simulink model "Noa_Nofusion"  (R2020b)
settings: Solver=FixedStepDiscrete  StartTime=0.0  StopTime=Inf  FixedStep=0.01  RelTol=1e-3
PostLoadFcn:
  | if any(exist('dsrtsu_mdlpostloadfcn', 'file') ~= 0), dsrtsu_mdlpostloadfcn('Execute', bdroot); end
InitFcn:
  | , if any(exist('rtifpga_mdlclblib', 'file') ~= 0), rtifpga_mdlclblib('Init', bdroot); end,
  | , if any(exist('dsmpb_private', 'file') ~= 0), dsmpb_private('dsmpb_mdlclblib', 'Init', bdroot); end,
undefined symbols (not defined in the file or in its folder): ACC_TimeGap_DecSetSwt, ACC_TimeGap_IncSetSwt, AccelPedalPosn, AccelPedalPosnVldty, AccelPedlPosnDiagc, AccPedalOverride, ACU_ShiftInProgress, ADAS_Posn_CurLane, AESSwtReq, ALC_SwtReq, BrkPedalSts, CC_ACC_CANCEL_OFFSwt, CC_ACC_CRUISE_OFFSwt, CC_ACC_DecSetSpd_SetSwt, CC_ACC_IncSetSpd_ResuSwt, CC_ACCSwtErr, CharSpd_ms, CSA_NODE, CURRENT_GEAR, CurrentGearValid, DiscIntNeverNeededParam, DrvDoorSts, DrvSBR, DrvTrqReqOvld, ECMACCInterface, ECMRespACC, ELKSwtReq, EngLimpHomeSts, EngSpd, EngState, EngState_PHEV, EngTrqMaxActSpd, EngTrqMinAct, EPS_DrvInpTrqVal_HighReslolution, EPS_FailSts, EPS_LKATorqOvrlDlvd, EPS_LKATorqOvrlDlvdVld, EPS_LKATrqOvlDlvdSts, EPS_SteerMod, EPS_TrqSnsrSts, EQ4_APPINFO, EQ4_LA_ELEM, EQ4_LA_HDR, EQ4_LAP_ELEM, EQ4_LAP_HDR, EQ4_LH_ELEM, EQ4_LH_HDR, EQ4_LRE_ELEM, EQ4_LRE_HDR, ESS_PedSwtReq, ESS_VehSwtReq, FFogLmpSts_F_Pbox, FLWheelDriveDirection, FLWheelSpd, FrntWiprSwtSts, FrntWshrSwtSts, FRWheelDriveDirection, FRWheelSpd, HazardLmpSwtSts, HCU_AccelPedalPosn_Diag ... (+151)
libraries: simulink x144, dsmpblib x33, canfdmsglib x10
(part 13 of 20)

== system Noa_Nofusion/Common/Subsystem7/DS/DriverStsConditnJudge/DSMidHi1Hi22NoDistractnJudge ==
  note: %Note
      | In order to cover one case at which distraction is no distraction but drowsns is low/middle/high 1/high2,add this
      | transition from low/middle/high 1/high2 distraction to no distraction.Conditions as follow:
      | DMSSts_ACC is 0x02: Active
      | && HeadDetn is 0x01: Yes
      | && DistrctnLevel_ACC is 0x00: No distraction
      | && DistrctnQlty_ACC≥ 85%
      | && During time is same as time of other to good
  canDMSSts : Inport
  canHeadDetn : Inport  Port=2
  canDistrctnLevel : Inport  Port=3
  canDistrctnQlty : Inport  Port=4
  Compare To Constant : simulink/Logic and Bit Operations/Compare To Constant  relop===  const=2  OutDataTypeStr=boolean
  Compare To Constant1 : simulink/Logic and Bit Operations/Compare To Constant  relop===  const=1  OutDataTypeStr=boolean
  Compare To Constant2 : simulink/Logic and Bit Operations/Compare To Constant  relop===  const=0  OutDataTypeStr=boolean
  Compare To Constant4 : simulink/Logic and Bit Operations/Compare To Constant  relop=>=  const=85  OutDataTypeStr=boolean
  Compare To Constant5 : simulink/Logic and Bit Operations/Compare To Constant  relop=>=  const=0.5  OutDataTypeStr=boolean
  Compare To Constant8 : simulink/Logic and Bit Operations/Compare To Constant  relop=<=  const=100  OutDataTypeStr=boolean
  Data Type Conversion : DataTypeConversion  OutDataTypeStr=single
  Logical Operator : Logic  Inputs=5  AllPortsSameDT=off  OutDataTypeStr=boolean
  counter : DiscreteIntegrator  ExternalReset=either  SampleTime=-1  LimitOutput=on  UpperSaturationLimit=10  LowerSaturationLimit=-10  ICPrevOutput=DiscIntNeverNeededParam  ICPrevScaledInput=DiscIntNeverNeededParam
  DSMidHi1Hi22NoDistractn : Outport
  wires:
  Compare To Constant5/1 -> DSMidHi1Hi22NoDistractn/1
  Compare To Constant8/1 -> Logical Operator/5
  Compare To Constant4/1 -> Logical Operator/4
  Compare To Constant2/1 -> Logical Operator/3
  Compare To Constant/1 -> Logical Operator/1
  Compare To Constant1/1 -> Logical Operator/2
  canDistrctnQlty/1 -> Compare To Constant4/1, Compare To Constant8/1
  counter/1 -> Compare To Constant5/1
  Logical Operator/1 -> Data Type Conversion/1
  canDistrctnLevel/1 -> Compare To Constant2/1
  canHeadDetn/1 -> Compare To Constant1/1
  canDMSSts/1 -> Compare To Constant/1
  Data Type Conversion/1 -> counter/2, counter/1

== system Noa_Nofusion/Common/Subsystem7/DS/DriverStsConditnJudge/DSMidHi1Hi22NoDrowsnsJudge ==
  note: %Note
      | In order to cover one case at which drowsns is no drowsiness but distraction is low/middle/high 1/high2,add this
      | transition from low/middle/high 1/high2 drowsiness to no drowsiness.Conditions as follow:
      | DMSSts_ACC is 0x02: Active
      | && HeadDetn is 0x01: Yes
      | && DrowsnsLevel_ACC is：0x0: No Drowsiness
      | && DrowsnsQlty_ACC≥85%
      | && During time is same as time of other to good
  canDMSSts : Inport
  canHeadDetn : Inport  Port=2
  canDrowsnsLevel : Inport  Port=3
  Compare To Constant : simulink/Logic and Bit Operations/Compare To Constant  relop===  const=2  OutDataTypeStr=boolean
  Compare To Constant1 : simulink/Logic and Bit Operations/Compare To Constant  relop===  const=1  OutDataTypeStr=boolean
  Compare To Constant2 : simulink/Logic and Bit Operations/Compare To Constant  relop===  const=0  OutDataTypeStr=boolean
  Compare To Constant5 : simulink/Logic and Bit Operations/Compare To Constant  relop=>=  const=0.5  OutDataTypeStr=boolean
  Data Type Conversion : DataTypeConversion  OutDataTypeStr=single
  Logical Operator : Logic  Inputs=3  AllPortsSameDT=off  OutDataTypeStr=boolean
  counter : DiscreteIntegrator  ExternalReset=either  SampleTime=-1  LimitOutput=on  UpperSaturationLimit=10  LowerSaturationLimit=-10  ICPrevOutput=DiscIntNeverNeededParam  ICPrevScaledInput=DiscIntNeverNeededParam
  DSMidHi1Hi22NoDrowsns : Outport
  wires:
  canDMSSts/1 -> Compare To Constant/1
  canHeadDetn/1 -> Compare To Constant1/1
  canDrowsnsLevel/1 -> Compare To Constant2/1
  Logical Operator/1 -> Data Type Conversion/1
  counter/1 -> Compare To Constant5/1
  Compare To Constant1/1 -> Logical Operator/2
  Compare To Constant/1 -> Logical Operator/1
  Compare To Constant2/1 -> Logical Operator/3
  Compare To Constant5/1 -> DSMidHi1Hi22NoDrowsns/1
  Data Type Conversion/1 -> counter/2, counter/1

== system Noa_Nofusion/Common/Subsystem7/DS/DriverStsConditnJudge/DSOther2GoodJudge ==
  note: %Note
      | Conditions of distraction state from Unbelievable∥Low∥Middle∥High Level 1∥High Level 2 to Good as follows:
      | DMSSts_ACC is 0x02: Active
      | && HeadDetn is 0x01: Yes
      | && DistrctnLevel_ACC is 0x00: No distraction
      | && DistrctnQlty_ACC≥ 85%
      | && DrowsnsLevel_ACC is：0x0: No Drowsiness
      | && DrowsnsQlty_ACC≥85%
      | && During time≥0.5s
  canDMSSts : Inport
  canHeadDetn : Inport  Port=2
  canDistrctnLevel : Inport  Port=3
  canDistrctnQlty : Inport  Port=4
  canDrowsnsLevel : Inport  Port=5
  Compare To Constant : simulink/Logic and Bit Operations/Compare To Constant  relop===  const=2  OutDataTypeStr=boolean
  Compare To Constant1 : simulink/Logic and Bit Operations/Compare To Constant  relop===  const=1  OutDataTypeStr=boolean
  Compare To Constant2 : simulink/Logic and Bit Operations/Compare To Constant  relop===  const=0  OutDataTypeStr=boolean
  Compare To Constant3 : simulink/Logic and Bit Operations/Compare To Constant  relop=>=  const=85  OutDataTypeStr=boolean
  Compare To Constant4 : simulink/Logic and Bit Operations/Compare To Constant  relop=<=  const=100  OutDataTypeStr=boolean
  Compare To Constant5 : simulink/Logic and Bit Operations/Compare To Constant  relop=>=  const=0.5  OutDataTypeStr=boolean
  Compare To Constant6 : simulink/Logic and Bit Operations/Compare To Constant  relop===  const=0  OutDataTypeStr=boolean
  Data Type Conversion : DataTypeConversion  OutDataTypeStr=single
  Logical Operator : Logic  Inputs=6  AllPortsSameDT=off  OutDataTypeStr=boolean
  counter : DiscreteIntegrator  ExternalReset=either  SampleTime=-1  LimitOutput=on  UpperSaturationLimit=10  LowerSaturationLimit=-10  ICPrevOutput=DiscIntNeverNeededParam  ICPrevScaledInput=DiscIntNeverNeededParam
  DSOther2Good : Outport
  wires:
  canDMSSts/1 -> Compare To Constant/1
  canHeadDetn/1 -> Compare To Constant1/1
  canDistrctnLevel/1 -> Compare To Constant2/1
  canDistrctnQlty/1 -> Compare To Constant4/1, Compare To Constant3/1
  Logical Operator/1 -> Data Type Conversion/1
  counter/1 -> Compare To Constant5/1
  canDrowsnsLevel/1 -> Compare To Constant6/1
  Compare To Constant/1 -> Logical Operator/1
  Compare To Constant1/1 -> Logical Operator/2
  Compare To Constant2/1 -> Logical Operator/3
  Compare To Constant3/1 -> Logical Operator/4
  Compare To Constant4/1 -> Logical Operator/5
  Compare To Constant6/1 -> Logical Operator/6
  Compare To Constant5/1 -> DSOther2Good/1
  Data Type Conversion/1 -> counter/2, counter/1

== system Noa_Nofusion/Common/Subsystem7/DS/DriverStsConditnJudge/DSOther2Hi1DistractnJudge ==
  note: %Note
      | Conditions of distraction state from other state to High 1 as follow:
      | DMSSts_ACC is 0x02: Active
      | && HeadDetn is 0x01: Yes
      | && DistrctnLevel_ACC is 0x03: Hi level distraction
      | && DistrctnQlty_ACC≥ 85%
      | && During time≥2s(adjustable)
  canDMSSts : Inport
  canHeadDetn : Inport  Port=2
  canDistrctnLevel : Inport  Port=3
  canDistrctnQlty : Inport  Port=4
  PtDSOther2Hi1Distractn : Inport  Port=5
  Compare To Constant : simulink/Logic and Bit Operations/Compare To Constant  relop===  const=2  OutDataTypeStr=boolean
  Compare To Constant1 : simulink/Logic and Bit Operations/Compare To Constant  relop===  const=1  OutDataTypeStr=boolean
  Compare To Constant2 : simulink/Logic and Bit Operations/Compare To Constant  relop===  const=3  OutDataTypeStr=boolean
  Compare To Constant4 : simulink/Logic and Bit Operations/Compare To Constant  relop=>=  const=85  OutDataTypeStr=boolean
  Compare To Constant8 : simulink/Logic and Bit Operations/Compare To Constant  relop=<=  const=100  OutDataTypeStr=boolean
  Data Type Conversion : DataTypeConversion  OutDataTypeStr=single
  Logical Operator : Logic  Inputs=5  AllPortsSameDT=off  OutDataTypeStr=boolean
  Relational Operator : RelationalOperator  OutDataTypeStr=boolean  RndMeth=Simplest
  counter : DiscreteIntegrator  ExternalReset=either  SampleTime=-1  LimitOutput=on  UpperSaturationLimit=10  LowerSaturationLimit=-10  ICPrevOutput=DiscIntNeverNeededParam  ICPrevScaledInput=DiscIntNeverNeededParam
  DSOther2Hi1Distractn : Outport
  wires:
  Logical Operator/1 -> Data Type Conversion/1
  canDMSSts/1 -> Compare To Constant/1
  canHeadDetn/1 -> Compare To Constant1/1
  canDistrctnLevel/1 -> Compare To Constant2/1
  canDistrctnQlty/1 -> Compare To Constant8/1, Compare To Constant4/1
  Compare To Constant1/1 -> Logical Operator/2
  Compare To Constant/1 -> Logical Operator/1
  Compare To Constant2/1 -> Logical Operator/3
  Compare To Constant4/1 -> Logical Operator/4
  Compare To Constant8/1 -> Logical Operator/5
  Relational Operator/1 -> DSOther2Hi1Distractn/1
  counter/1 -> Relational Operator/1
  PtDSOther2Hi1Distractn/1 -> Relational Operator/2
  Data Type Conversion/1 -> counter/2, counter/1

== system Noa_Nofusion/Common/Subsystem7/DS/DriverStsConditnJudge/DSOther2Hi1DrowsnsJudge ==
  note: %Note
      | Conditions of drowsns state from other state to High 1 as follow:
      | DMSSts_ACC is 0x02: Active
      | && HeadDetn is 0x01: Yes
      | && DrowsnsLevel_ACC is 0x3: Hi level Drowsiness
      | && DrowsnsQlty_ACC≥85%
      | && During time≥0.5s(adjustable)
  canDMSSts : Inport
  canHeadDetn : Inport  Port=2
  canDrowsnsLevel : Inport  Port=3
  PtDSOther2Hi1Drowsns : Inport  Port=4
  Compare To Constant : simulink/Logic and Bit Operations/Compare To Constant  relop===  const=2  OutDataTypeStr=boolean
  Compare To Constant1 : simulink/Logic and Bit Operations/Compare To Constant  relop===  const=1  OutDataTypeStr=boolean
  Compare To Constant2 : simulink/Logic and Bit Operations/Compare To Constant  relop===  const=3  OutDataTypeStr=boolean
  Data Type Conversion : DataTypeConversion  OutDataTypeStr=single
  Logical Operator : Logic  Inputs=3  AllPortsSameDT=off  OutDataTypeStr=boolean
  Relational Operator : RelationalOperator  OutDataTypeStr=boolean  RndMeth=Simplest
  counter : DiscreteIntegrator  ExternalReset=either  SampleTime=-1  LimitOutput=on  UpperSaturationLimit=10  LowerSaturationLimit=-10  ICPrevOutput=DiscIntNeverNeededParam  ICPrevScaledInput=DiscIntNeverNeededParam
  DSOther2Hi1Drowsns : Outport
  wires:
  counter/1 -> Relational Operator/1
  Relational Operator/1 -> DSOther2Hi1Drowsns/1
  Compare To Constant2/1 -> Logical Operator/3
  Compare To Constant/1 -> Logical Operator/1
  Compare To Constant1/1 -> Logical Operator/2
  canDrowsnsLevel/1 -> Compare To Constant2/1
  canHeadDetn/1 -> Compare To Constant1/1
  canDMSSts/1 -> Compare To Constant/1
  Logical Operator/1 -> Data Type Conversion/1
  PtDSOther2Hi1Drowsns/1 -> Relational Operator/2
  Data Type Conversion/1 -> counter/2, counter/1

== system Noa_Nofusion/Common/Subsystem7/DS/DriverStsConditnJudge/DSOther2Hi2DistractnJudge ==
  note: %Note
      | Conditions of distraction state from other state to High 2 as follow:
      | DMSSts_ACC is 0x02: Active
      | && HeadDetn is 0x01: Yes
      | && DistrctnLevel_ACC is 0x03: Hi level distraction
      | && DistrctnQlty_ACC≥ 85%
      | && During time≥5s(adjustable)
  canDMSSts : Inport
  canHeadDetn : Inport  Port=2
  canDistrctnLevel : Inport  Port=3
  canDistrctnQlty : Inport  Port=4
  PtDSOther2Hi2Distractn : Inport  Port=5
  Compare To Constant : simulink/Logic and Bit Operations/Compare To Constant  relop===  const=2  OutDataTypeStr=boolean
  Compare To Constant1 : simulink/Logic and Bit Operations/Compare To Constant  relop===  const=1  OutDataTypeStr=boolean
  Compare To Constant2 : simulink/Logic and Bit Operations/Compare To Constant  relop===  const=3  OutDataTypeStr=boolean
  Compare To Constant4 : simulink/Logic and Bit Operations/Compare To Constant  relop=>=  const=85  OutDataTypeStr=boolean
  Compare To Constant8 : simulink/Logic and Bit Operations/Compare To Constant  relop=<=  const=100  OutDataTypeStr=boolean
  Data Type Conversion : DataTypeConversion  OutDataTypeStr=single
  Logical Operator : Logic  Inputs=5  AllPortsSameDT=off  OutDataTypeStr=boolean
  Relational Operator : RelationalOperator  OutDataTypeStr=boolean  RndMeth=Simplest
  counter : DiscreteIntegrator  ExternalReset=either  SampleTime=-1  LimitOutput=on  UpperSaturationLimit=10  LowerSaturationLimit=-10  ICPrevOutput=DiscIntNeverNeededParam  ICPrevScaledInput=DiscIntNeverNeededParam
  DSOther2Hi2Distractn : Outport
  wires:
  counter/1 -> Relational Operator/1
  Relational Operator/1 -> DSOther2Hi2Distractn/1
  Compare To Constant8/1 -> Logical Operator/5
  Compare To Constant4/1 -> Logical Operator/4
  Compare To Constant2/1 -> Logical Operator/3
  Compare To Constant/1 -> Logical Operator/1
  Compare To Constant1/1 -> Logical Operator/2
  canDistrctnQlty/1 -> Compare To Constant4/1, Compare To Constant8/1
  canDistrctnLevel/1 -> Compare To Constant2/1
  canHeadDetn/1 -> Compare To Constant1/1
  canDMSSts/1 -> Compare To Constant/1
  Logical Operator/1 -> Data Type Conversion/1
  PtDSOther2Hi2Distractn/1 -> Relational Operator/2
  Data Type Conversion/1 -> counter/2, counter/1

== system Noa_Nofusion/Common/Subsystem7/DS/DriverStsConditnJudge/DSOther2Hi2DrowsnsJudge ==
  note: %Note
      | Conditions of drowsns state from other state to High2 as follow:
      | DMSSts_ACC is 0x02: Active
      | && HeadDetn is 0x01: Yes
      | && DrowsnsLevel_ACC is 0x3: Hi level Drowsiness
      | && DrowsnsQlty_ACC≥85%
      | && During time≥3s(adjustable)
  canDMSSts : Inport
  canHeadDetn : Inport  Port=2
  canDrowsnsLevel : Inport  Port=3
  PtDSOther2Hi2Drowsns : Inport  Port=4
  Compare To Constant : simulink/Logic and Bit Operations/Compare To Constant  relop===  const=2  OutDataTypeStr=boolean
  Compare To Constant1 : simulink/Logic and Bit Operations/Compare To Constant  relop===  const=1  OutDataTypeStr=boolean
  Compare To Constant2 : simulink/Logic and Bit Operations/Compare To Constant  relop===  const=3  OutDataTypeStr=boolean
  Data Type Conversion : DataTypeConversion  OutDataTypeStr=single
  Logical Operator : Logic  Inputs=3  AllPortsSameDT=off  OutDataTypeStr=boolean
  Relational Operator : RelationalOperator  OutDataTypeStr=boolean  RndMeth=Simplest
  counter : DiscreteIntegrator  ExternalReset=either  SampleTime=-1  LimitOutput=on  UpperSaturationLimit=10  LowerSaturationLimit=-10  ICPrevOutput=DiscIntNeverNeededParam  ICPrevScaledInput=DiscIntNeverNeededParam
  DSOther2Hi2Drowsns : Outport
  wires:
  Logical Operator/1 -> Data Type Conversion/1
  canDMSSts/1 -> Compare To Constant/1
  canHeadDetn/1 -> Compare To Constant1/1
  canDrowsnsLevel/1 -> Compare To Constant2/1
  Relational Operator/1 -> DSOther2Hi2Drowsns/1
  Compare To Constant1/1 -> Logical Operator/2
  Compare To Constant/1 -> Logical Operator/1
  Compare To Constant2/1 -> Logical Operator/3
  counter/1 -> Relational Operator/1
  PtDSOther2Hi2Drowsns/1 -> Relational Operator/2
  Data Type Conversion/1 -> counter/2, counter/1

== system Noa_Nofusion/Common/Subsystem7/DS/DriverStsConditnJudge/DSOther2UnbelivJudge ==
  note: %Note
      | Conditions of distraction and drowsns state from other to unbelievable as follow:
      | (DMSSts_ACC is no 0x02: Active&& during time ≥3cycles)
      | ∥ (HeadDetn is 0x00: No&&during time≥3s)
      | ∥(DistrctnLevel_ACC is 0x7: Invalid &&during time≥3s)
      | ∥(DrowsnsLevel_ACC is 0x7: Invalid &&during time≥3s)
      | ∥{DistrctnQlty_ACC is 0x7F:Invalid data &&during time≥3s}
      | ∥{DrowsnsQlty_ACC is 0x7F:Invalid data &&during time≥3s}
  canDMSSts : Inport
  canHeadDetn : Inport  Port=2
  canDistrctnLevel : Inport  Port=3
  canDistrctnQlty : Inport  Port=4
  canDrowsnsLevel : Inport  Port=5
  Compare To Constant : simulink/Logic and Bit Operations/Compare To Constant  relop=~=  const=2  OutDataTypeStr=boolean
  Compare To Constant1 : simulink/Logic and Bit Operations/Compare To Constant  relop===  const=0  OutDataTypeStr=boolean
  Compare To Constant{4,9..11} (4 alike) : simulink/Logic and Bit Operations/Compare To Constant  relop=>=  const=3  OutDataTypeStr=boolean
  Compare To Constant2 : simulink/Logic and Bit Operations/Compare To Constant  relop===  const=7  OutDataTypeStr=boolean
  Compare To Constant3 : simulink/Logic and Bit Operations/Compare To Constant  relop===  const=127  OutDataTypeStr=boolean
  Compare To Constant6 : simulink/Logic and Bit Operations/Compare To Constant  relop===  const=7  OutDataTypeStr=boolean
  Data Type Conversion{,1..4} (5 alike) : DataTypeConversion  OutDataTypeStr=single
  Logical Operator : Logic  Operator=OR  Inputs=5  AllPortsSameDT=off  OutDataTypeStr=boolean
  counter{,1..4} (5 alike) : DiscreteIntegrator  ExternalReset=either  SampleTime=-1  LimitOutput=on  UpperSaturationLimit=10  LowerSaturationLimit=-10  ICPrevOutput=DiscIntNeverNeededParam  ICPrevScaledInput=DiscIntNeverNeededParam
  tCycle3plus : simulink/Logic and Bit Operations/Compare To Constant  relop=>=  const=0.06  OutDataTypeStr=boolean
  DSOther2Unbeliv : Outport
  wires:
  Logical Operator/1 -> DSOther2Unbeliv/1
  canDrowsnsLevel/1 -> Compare To Constant6/1
  canDistrctnQlty/1 -> Compare To Constant3/1
  canDistrctnLevel/1 -> Compare To Constant2/1
  canHeadDetn/1 -> Compare To Constant1/1
  canDMSSts/1 -> Compare To Constant/1
  Compare To Constant1/1 -> Data Type Conversion1/1
  Compare To Constant2/1 -> Data Type Conversion2/1
  Compare To Constant6/1 -> Data Type Conversion3/1
  Compare To Constant3/1 -> Data Type Conversion4/1
  Compare To Constant10/1 -> Logical Operator/3
  Compare To Constant11/1 -> Logical Operator/4
  Compare To Constant9/1 -> Logical Operator/2
  Compare To Constant4/1 -> Logical Operator/5
  tCycle3plus/1 -> Logical Operator/1
  Compare To Constant/1 -> Data Type Conversion/1
  counter/1 -> tCycle3plus/1
  counter1/1 -> Compare To Constant9/1
  counter2/1 -> Compare To Constant10/1
  counter3/1 -> Compare To Constant11/1
  counter4/1 -> Compare To Constant4/1
  Data Type Conversion/1 -> counter/2, counter/1
  Data Type Conversion1/1 -> counter1/2, counter1/1
  Data Type Conversion2/1 -> counter2/2, counter2/1
  Data Type Conversion3/1 -> counter3/2, counter3/1
  Data Type Conversion4/1 -> counter4/2, counter4/1

== system Noa_Nofusion/Common/Subsystem7/DS/DriverStsConditnJudge/DSUnbeliv2DDAJudge ==
  note: %Note
      | Following condition aims to prevent transition between DDA and Unbelievable constantly
      | DMSSts_ACC is 0x02: Active&&
      | HeadDetn is 0x01: Yes &&
      | DistrctnLevel_ACC is no 0x7: Invalid&&
      | DrowsnsLevel_ACC is no 0x7: Invalid&&
      | DistrctnQlty_ACC is no 0x7F:Invalid&&
      | DrowsnsQlty_ACC is no 0x7F:Invalid
  canDMSSts : Inport
  canHeadDetn : Inport  Port=2
  canDistrctnLevel : Inport  Port=3
  canDistrctnQlty : Inport  Port=4
  canDrowsnsLevel : Inport  Port=5
  Compare To Constant : simulink/Logic and Bit Operations/Compare To Constant  relop===  const=2  OutDataTypeStr=boolean
  Compare To Constant1 : simulink/Logic and Bit Operations/Compare To Constant  relop===  const=1  OutDataTypeStr=boolean
  Compare To Constant2 : simulink/Logic and Bit Operations/Compare To Constant  relop=~=  const=7  OutDataTypeStr=boolean
  Compare To Constant3 : simulink/Logic and Bit Operations/Compare To Constant  relop=~=  const=127  OutDataTypeStr=boolean
  Compare To Constant6 : simulink/Logic and Bit Operations/Compare To Constant  relop=~=  const=7  OutDataTypeStr=boolean
  Logical Operator : Logic  Inputs=5  AllPortsSameDT=off  OutDataTypeStr=boolean
  DSUnbeliv2DDAEnable : Outport
  wires:
  canDMSSts/1 -> Compare To Constant/1
  canHeadDetn/1 -> Compare To Constant1/1
  canDistrctnLevel/1 -> Compare To Constant2/1
  canDistrctnQlty/1 -> Compare To Constant3/1
  canDrowsnsLevel/1 -> Compare To Constant6/1
  Logical Operator/1 -> DSUnbeliv2DDAEnable/1
  Compare To Constant/1 -> Logical Operator/1
  Compare To Constant1/1 -> Logical Operator/2
  Compare To Constant2/1 -> Logical Operator/3
  Compare To Constant6/1 -> Logical Operator/4
  Compare To Constant3/1 -> Logical Operator/5

== system Noa_Nofusion/TOS/Subsystem2/ACCOSM/HWA_Task100ms1/OTL1 ==
  vRef : Inport
  tCycle : Inport  Port=2
  tSameHandle : Inport  Port=3
  CutIn : Inport  Port=4
  P0Dx : Inport  Port=5
  P0Dy : Inport  Port=6
  EgoDDeltaX : Inport  Port=7
  EgoDDeltaY : Inport  Port=8
  EgoCosOfPsi : Inport  Port=9
  EgoSinOfPsi : Inport  Port=10
  TarLineValid : Inport  Port=11
  TarLineA2 : Inport  Port=12
  TarLineA1 : Inport  Port=13
  TarLineA0 : Inport  Port=14
  Abs : Abs
  CutIn1 : InportShadow  Port=4
  Logical Operator : Logic  AllPortsSameDT=off  OutDataTypeStr=boolean
  Logical Operator1 : Logic  AllPortsSameDT=off  OutDataTypeStr=boolean
  MATLAB Function : MATLAB Function  TreatAsAtomicUnit=on
  Memory31 : Memory  InitialCondition=zeros(24,1)  InheritSampleTime=on
  Memory32 : Memory  InitialCondition=zeros(24,1)  InheritSampleTime=on
  Memory33 : Memory  InitialCondition=uint8(0)  InheritSampleTime=on
  P0TrajHistCalc01 : MATLAB Function  TreatAsAtomicUnit=on
  P0TrajHistCalc1 : MATLAB Function  TreatAsAtomicUnit=on
  Terminator : Terminator
  Terminator1 : Terminator
  Terminator2 : Terminator
  Unit Delay : UnitDelay  SampleTime=-1  HasFrameUpgradeWarning=on
  tSameHandle1 : InportShadow  Port=3
  LineValid : Outport
  a : Outport  Port=2
  b : Outport  Port=3
  c : Outport  Port=4
  d : Outport  Port=5
  dxMin : Outport  Port=6
  dxMax : Outport  Port=7
  wires:
  vRef/1 -> P0TrajHistCalc01/1(vRef)
  CutIn/1 -> P0TrajHistCalc01/4(CutIn)
  P0TrajHistCalc1/8(d) -> d/1
  P0TrajHistCalc1/10(dxMax) -> dxMax/1
  P0TrajHistCalc1/9(dxMin) -> dxMin/1
  P0TrajHistCalc1/7(c) -> c/1
  P0TrajHistCalc1/6(b) -> b/1
  P0TrajHistCalc1/5(a) -> a/1
  P0TrajHistCalc1/4(LineValid) -> Logical Operator/2
  P0TrajHistCalc1/3(P0TrajHistDyv) -> Terminator2/1
  P0TrajHistCalc1/2(P0TrajHistDxv) -> Terminator1/1
  P0TrajHistCalc1/1(P0TrajHistNum) -> Terminator/1
  P0Dy/1 -> P0TrajHistCalc01/6(P0Dy)
  P0Dx/1 -> P0TrajHistCalc01/5(P0Dx)
  tSameHandle/1 -> P0TrajHistCalc01/3(tSameHandle)
  EgoCosOfPsi/1 -> P0TrajHistCalc01/9(EgoCosOfPsi)
  tCycle/1 -> P0TrajHistCalc01/2(tCycle)
  Memory31/1 -> P0TrajHistCalc01/17(P0TrajHistDyvK1)
  EgoDDeltaY/1 -> P0TrajHistCalc01/8(EgoDDeltaY)
  P0TrajHistCalc01/3(P0TrajHistDxv) -> P0TrajHistCalc1/2(P0TrajHistDxv1), Memory32/1
  Memory32/1 -> P0TrajHistCalc01/16(P0TrajHistDxvK1)
  P0TrajHistCalc01/2(P0TrajHistNum) -> P0TrajHistCalc1/1(P0TrajHistNum1), Memory33/1
  EgoSinOfPsi/1 -> P0TrajHistCalc01/10(EgoSinOfPsi)
  Memory33/1 -> P0TrajHistCalc01/15(P0TrajHistNumK1)
  P0TrajHistCalc01/4(P0TrajHistDyv) -> P0TrajHistCalc1/3(P0TrajHistDyv1), Memory31/1
  EgoDDeltaX/1 -> P0TrajHistCalc01/7(EgoDDeltaX)
  TarLineValid/1 -> P0TrajHistCalc01/11(TarLineValid)
  TarLineA2/1 -> P0TrajHistCalc01/12(TarLineA2)
  TarLineA1/1 -> P0TrajHistCalc01/13(TarLineA1)
  TarLineA0/1 -> P0TrajHistCalc01/14(TarLineA0)
  tSameHandle1/1 -> MATLAB Function/1(t)
  CutIn1/1 -> Logical Operator1/1
  MATLAB Function/1(Valid) -> Logical Operator/1, Unit Delay/1
  Unit Delay/1 -> MATLAB Function/3(ValidK1)
  Logical Operator/1 -> LineValid/1
  P0TrajHistCalc01/1(P0Dyc) -> Abs/1
  Abs/1 -> Logical Operator1/2
  Logical Operator1/1 -> MATLAB Function/2(CutIn_b)

== system Noa_Nofusion/TOS/Subsystem2/ACCOSM/HWA_Task100ms1/Trajectory ==
  Kap : Inport
  VxvRef : Inport  Port=2
  AlpSideSlipAngle : Inport  Port=3
  ObjValid : Inport  Port=4
  ObjDx : Inport  Port=5
  ObjDy : Inport  Port=6
  ObjClass : Inport  Port=7
  ObjCntAlive : Inport  Port=8
  Terminator{1,3..10} (9 alike) : Terminator
  Trajectory : Subsystem  mask{ObjNum=15, TrajNum=10, BufNum=24}
      mask prompts: ObjNum "ObjectNumber"; TrajNum "TrajectoryNumber"; BufNum "BufferNumber"
  Out8 : Outport
  Out9 : Outport  Port=2
  Out10 : Outport  Port=3
  Out11 : Outport  Port=4
  Out12 : Outport  Port=5
  Out13 : Outport  Port=6
  EgoMove : Outport  Port=7
  wires:
  Trajectory/16(EgoMove) -> EgoMove/1
  Trajectory/11(TrajHistBufferBValid) -> Out11/1
  Trajectory/12(TrajHistBufferDxv) -> Out12/1
  Trajectory/13(TrajHistBufferDyv) -> Out13/1
  ObjValid/1 -> Trajectory/4(ObjValid)
  ObjDx/1 -> Trajectory/5(ObjectDx)
  ObjDy/1 -> Trajectory/6(ObjectDy)
  ObjClass/1 -> Trajectory/7(ObjectClass)
  ObjCntAlive/1 -> Trajectory/8(ObjectCntAlive)
  Kap/1 -> Trajectory/1(KapTraj)
  Trajectory/8(TrajHistBufferBTrajEnd) -> Out8/1
  Trajectory/2(EgoTrajHistDxv) -> Terminator4/1
  Trajectory/5(ObjPrio) -> Terminator8/1
  Trajectory/1(EgoTrajHistCurrentIndex) -> Terminator3/1
  AlpSideSlipAngle/1 -> Trajectory/3(AlpSideSlipAngle)
  Trajectory/7(TrajUsed) -> Terminator9/1
  Trajectory/10(TrajCurrentIndex) -> Out10/1
  Trajectory/6(ObjMatrix) -> Terminator10/1
  Trajectory/4(EgoTrajHistTTimeStamp) -> Terminator7/1
  VxvRef/1 -> Trajectory/2(VxvRef)
  Trajectory/3(EgoTrajHistDyv) -> Terminator5/1
  Trajectory/9(ObjTrajNumber) -> Out9/1
  Trajectory/14(TrajHistBufferTTimeStamp) -> Terminator6/1
  Trajectory/15(TrajHistBufferClass) -> Terminator1/1

== system Noa_Nofusion/TOS/Subsystem2/ACCOSM/HWA_Task100ms1/VxVy ==
  VxvRef : Inport
  Kap : Inport  Port=2
  VxG : Inport  Port=3
  VyG : Inport  Port=4
  Constant2 : Constant  Value=P_Global_EQ2RearAxisX_m  OutDataTypeStr=single
  Constant4 : Constant  Value=SideSlipAnglefactor  OutDataTypeStr=single
  Divide11 : Product
  Divide3 : Product  Inputs=3
  Divide4 : Product
  Divide5 : Product
  Gain10 : Gain  Gain=-1
  Gain9 : Gain  Gain=-1
  Sum1 : Sum  Inputs=+-
  Sum10 : Sum  Inputs=+-|
  Sum11 : Sum  Inputs=|-+
  Trigonometric Function : Trigonometry  Operator=atan  OutputSignalType=real
  Trigonometric Function1 : Trigonometry  Operator=cos
  Trigonometric Function2 : Trigonometry
  Vx : Outport
  Vy : Outport  Port=2
  wires:
  VxvRef/1 -> Divide3/2, Divide11/1, Divide5/1, Divide3/3
  Constant4/1 -> Divide3/1
  Trigonometric Function/1 -> Gain9/1
  Divide11/1 -> Sum11/1
  Constant2/1 -> Sum1/1
  Trigonometric Function1/1 -> Divide5/2
  Divide4/1 -> Trigonometric Function/1
  Divide5/1 -> Sum10/2
  Gain10/1 -> Trigonometric Function1/1, Trigonometric Function2/1
  Divide3/1 -> Sum1/2
  [IFVMoveAngle] -> Gain10/1
  Trigonometric Function2/1 -> Divide11/2
  Sum1/1 -> Divide4/1
  Gain9/1 -> [IFVMoveAngle]
  VxG/1 -> Sum10/1
  Sum11/1 -> Vy/1  "Vy"
  Sum10/1 -> Vx/1  "Vx"
  VyG/1 -> Sum11/2
  Kap/1 -> Divide4/2

== system Noa_Nofusion/TOS/Subsystem2/ACCOSM/ObjMatrixTransit/Subsystem ==
  Count : Inport
  <EQ4_OBJ_ELEM> : Inport  Port=2
  Bus Creator : BusCreator  Inputs=12
  Bus Selector : BusSelector  OutputSignals=id,BrakeLight,classification,LatDis,AbsLatVel,AbsLongAcc,LongDis,AbsLongVel,width,Age,motionSts
  For Each Subsystem : Subsystem  TreatAsAtomicUnit=on
  For Iterator Subsystem : Subsystem  Commented=on  TreatAsAtomicUnit=on
  MATLAB Function1 : MATLAB Function  TreatAsAtomicUnit=on
  Obj : Stateflow chart  Commented=on  TreatAsAtomicUnit=on
  Terminator : Terminator
  Terminator1 : Terminator
  Unit Delay1 : UnitDelay  SampleTime=-1  HasFrameUpgradeWarning=on
  ObjID : Outport
  ObjValid : Outport  Port=2
  ObjBrakeLightIndic : Outport  Port=3
  ObjClassification : Outport  Port=4
  ObjLatPos : Outport  Port=5
  ObjLatVel : Outport  Port=6
  ObjLongAccel : Outport  Port=7
  ObjLongVel : Outport  Port=8
  ObjWidth : Outport  Port=9
  ObjCnt : Outport  Port=10
  ObjMoveSts : Outport  Port=11
  ObjLongPos : Outport  Port=12
  P : Outport  Port=13
  ObjClass : Outport  Port=14
  wires:
  For Each Subsystem/6(LatDis) -> Bus Creator/6  "LatDis"
  Bus Creator/1 -> Bus Selector/1
  MATLAB Function1/14(ObjID) -> ObjID/1, Unit Delay1/1  "ObjBrakeLightIndic"
  For Each Subsystem/10(BrakeLight) -> Bus Creator/10  "BrakeLight"
  MATLAB Function1/6(ObjLatPos) -> ObjLatPos/1
  For Each Subsystem/7(AbsLongAcc) -> Bus Creator/7  "AbsLongAcc"
  For Each Subsystem/12(motionSts) -> Bus Creator/12  "motionSts"
  MATLAB Function1/5(ObjClassification) -> ObjClassification/1
  MATLAB Function1/8(ObjLongAccel) -> ObjLongAccel/1
  For Each Subsystem/14(motionOrientation) -> Terminator1/1
  Count/1 -> MATLAB Function1/1(Count)
  For Each Subsystem/8(AbsLongVel) -> Bus Creator/8  "AbsLongVel"
  For Each Subsystem/4(width) -> Bus Creator/4  "width"
  For Each Subsystem/13(motionCategory) -> Terminator/1
  For Each Subsystem/9(AbsLatVel) -> Bus Creator/9  "AbsLatVel"
  For Each Subsystem/5(LongDis) -> Bus Creator/5  "LongDis"
  Bus Selector/10 -> MATLAB Function1/11(Age)  "<Age>"
  For Each Subsystem/3(classification) -> Bus Creator/3  "classification"
  Bus Selector/8 -> MATLAB Function1/9(LongVel)  "<AbsLongVel>"
  Bus Selector/3 -> MATLAB Function1/4(Class)  "<classification>"
  For Each Subsystem/1(id) -> Bus Creator/1  "id"
  For Each Subsystem/11(Age) -> Bus Creator/11  "Age"
  For Each Subsystem/2(confidence) -> Bus Creator/2  "confidence"
  Bus Selector/7 -> MATLAB Function1/8(LongDis)  "<LongDis>"
  Bus Selector/9 -> MATLAB Function1/10(Width)  "<width>"
  Bus Selector/5 -> MATLAB Function1/6(LatVel)  "<AbsLatVel>"
  Bus Selector/6 -> MATLAB Function1/7(LongAccel)  "<AbsLongAcc>"
  Bus Selector/4 -> MATLAB Function1/5(LatDis)  "<LatDis>"
  MATLAB Function1/12(ObjMoveSts) -> ObjMoveSts/1
  Bus Selector/11 -> MATLAB Function1/12(MotionSts)  "<motionSts>"
  MATLAB Function1/13(ObjLongPos) -> ObjLongPos/1
  MATLAB Function1/1(P) -> P/1
  Bus Selector/2 -> MATLAB Function1/3(BrakeLight_b)  "<BrakeLight>"
  Bus Selector/1 -> MATLAB Function1/2(ID)  "<id>"
  Unit Delay1/1 -> MATLAB Function1/13(ObjIDK1)
  <EQ4_OBJ_ELEM>/1 -> For Each Subsystem/1(<EQ4_OBJ_ELEM>)
  MATLAB Function1/2(ObjValid) -> ObjValid/1
  MATLAB Function1/7(ObjLatVel) -> ObjLatVel/1
  MATLAB Function1/3(ObjBrakeLightIndic) -> ObjBrakeLightIndic/1
  MATLAB Function1/9(ObjLongVel) -> ObjLongVel/1
  MATLAB Function1/10(ObjWidth) -> ObjWidth/1
  MATLAB Function1/11(ObjCnt) -> ObjCnt/1
  MATLAB Function1/4(ObjClass) -> ObjClass/1

== system Noa_Nofusion/TOS/Subsystem2/DOP/HWA_Task100ms1/OTL1 ==
  vRef : Inport
  tCycle : Inport  Port=2
  tSameHandle : Inport  Port=3
  CutIn : Inport  Port=4
  P0Dx : Inport  Port=5
  P0Dy : Inport  Port=6
  EgoDDeltaX : Inport  Port=7
  EgoDDeltaY : Inport  Port=8
  EgoCosOfPsi : Inport  Port=9
  EgoSinOfPsi : Inport  Port=10
  TarLineValid : Inport  Port=11
  TarLineA2 : Inport  Port=12
  TarLineA1 : Inport  Port=13
  TarLineA0 : Inport  Port=14
  Memory31 : Memory  InitialCondition=zeros(24,1)  InheritSampleTime=on
  Memory32 : Memory  InitialCondition=zeros(24,1)  InheritSampleTime=on
  Memory33 : Memory  InitialCondition=uint8(0)  InheritSampleTime=on
  P0TrajHistCalc01 : MATLAB Function  TreatAsAtomicUnit=on
  P0TrajHistCalc1 : MATLAB Function  TreatAsAtomicUnit=on
  Terminator{,1..3} (4 alike) : Terminator
  LineValid : Outport
  a : Outport  Port=2
  b : Outport  Port=3
  c : Outport  Port=4
  d : Outport  Port=5
  dxMin : Outport  Port=6
  dxMax : Outport  Port=7
  wires:
  P0TrajHistCalc01/1(P0Dyc) -> Terminator3/1
  P0TrajHistCalc1/4(LineValid) -> LineValid/1
  TarLineA0/1 -> P0TrajHistCalc01/14(TarLineA0)
  TarLineA1/1 -> P0TrajHistCalc01/13(TarLineA1)
  TarLineA2/1 -> P0TrajHistCalc01/12(TarLineA2)
  TarLineValid/1 -> P0TrajHistCalc01/11(TarLineValid)
  EgoDDeltaX/1 -> P0TrajHistCalc01/7(EgoDDeltaX)
  P0TrajHistCalc01/4(P0TrajHistDyv) -> Memory31/1, P0TrajHistCalc1/3(P0TrajHistDyv1)
  Memory33/1 -> P0TrajHistCalc01/15(P0TrajHistNumK1)
  EgoSinOfPsi/1 -> P0TrajHistCalc01/10(EgoSinOfPsi)
  P0TrajHistCalc01/2(P0TrajHistNum) -> Memory33/1, P0TrajHistCalc1/1(P0TrajHistNum1)
  Memory32/1 -> P0TrajHistCalc01/16(P0TrajHistDxvK1)
  P0TrajHistCalc01/3(P0TrajHistDxv) -> Memory32/1, P0TrajHistCalc1/2(P0TrajHistDxv1)
  EgoDDeltaY/1 -> P0TrajHistCalc01/8(EgoDDeltaY)
  Memory31/1 -> P0TrajHistCalc01/17(P0TrajHistDyvK1)
  tCycle/1 -> P0TrajHistCalc01/2(tCycle)
  EgoCosOfPsi/1 -> P0TrajHistCalc01/9(EgoCosOfPsi)
  tSameHandle/1 -> P0TrajHistCalc01/3(tSameHandle)
  P0Dx/1 -> P0TrajHistCalc01/5(P0Dx)
  P0Dy/1 -> P0TrajHistCalc01/6(P0Dy)
  P0TrajHistCalc1/1(P0TrajHistNum) -> Terminator/1
  P0TrajHistCalc1/2(P0TrajHistDxv) -> Terminator1/1
  P0TrajHistCalc1/3(P0TrajHistDyv) -> Terminator2/1
  P0TrajHistCalc1/5(a) -> a/1
  P0TrajHistCalc1/6(b) -> b/1
  P0TrajHistCalc1/7(c) -> c/1
  P0TrajHistCalc1/9(dxMin) -> dxMin/1
  P0TrajHistCalc1/10(dxMax) -> dxMax/1
  P0TrajHistCalc1/8(d) -> d/1
  CutIn/1 -> P0TrajHistCalc01/4(CutIn)
  vRef/1 -> P0TrajHistCalc01/1(vRef)

== system Noa_Nofusion/TOS/Subsystem2/DOP/HWA_Task100ms1/Trajectory ==
  Kap : Inport
  VxvRef : Inport  Port=2
  AlpSideSlipAngle : Inport  Port=3
  ObjValid : Inport  Port=4
  ObjDx : Inport  Port=5
  ObjDy : Inport  Port=6
  ObjClass : Inport  Port=7
  ObjCntAlive : Inport  Port=8
  Terminator{1,3..10} (9 alike) : Terminator
  Trajectory : Subsystem  mask{ObjNum=15, TrajNum=10, BufNum=24}
      mask prompts: ObjNum "ObjectNumber"; TrajNum "TrajectoryNumber"; BufNum "BufferNumber"
  Out8 : Outport
  Out9 : Outport  Port=2
  Out10 : Outport  Port=3
  Out11 : Outport  Port=4
  Out12 : Outport  Port=5
  Out13 : Outport  Port=6
  EgoMove : Outport  Port=7
  wires:
  Trajectory/15(TrajHistBufferClass) -> Terminator1/1
  Trajectory/14(TrajHistBufferTTimeStamp) -> Terminator6/1
  Trajectory/9(ObjTrajNumber) -> Out9/1
  Trajectory/3(EgoTrajHistDyv) -> Terminator5/1
  VxvRef/1 -> Trajectory/2(VxvRef)
  Trajectory/4(EgoTrajHistTTimeStamp) -> Terminator7/1
  Trajectory/6(ObjMatrix) -> Terminator10/1
  Trajectory/10(TrajCurrentIndex) -> Out10/1
  Trajectory/7(TrajUsed) -> Terminator9/1
  AlpSideSlipAngle/1 -> Trajectory/3(AlpSideSlipAngle)
  Trajectory/1(EgoTrajHistCurrentIndex) -> Terminator3/1
  Trajectory/5(ObjPrio) -> Terminator8/1
  Trajectory/2(EgoTrajHistDxv) -> Terminator4/1
  Trajectory/8(TrajHistBufferBTrajEnd) -> Out8/1
  Kap/1 -> Trajectory/1(KapTraj)
  ObjCntAlive/1 -> Trajectory/8(ObjectCntAlive)
  ObjClass/1 -> Trajectory/7(ObjectClass)
  ObjDy/1 -> Trajectory/6(ObjectDy)
  ObjDx/1 -> Trajectory/5(ObjectDx)
  ObjValid/1 -> Trajectory/4(ObjValid)
  Trajectory/13(TrajHistBufferDyv) -> Out13/1
  Trajectory/12(TrajHistBufferDxv) -> Out12/1
  Trajectory/11(TrajHistBufferBValid) -> Out11/1
  Trajectory/16(EgoMove) -> EgoMove/1

== system Noa_Nofusion/TOS/Subsystem2/DOP/HWA_Task100ms1/VxVy ==
  VxvRef : Inport
  Kap : Inport  Port=2
  VxG : Inport  Port=3
  VyG : Inport  Port=4
  Constant2 : Constant  Value=P_Global_EQ2RearAxisX_m  OutDataTypeStr=single
  Constant4 : Constant  Value=SideSlipAnglefactor  OutDataTypeStr=single
  Divide11 : Product
  Divide3 : Product  Inputs=3
  Divide4 : Product
  Divide5 : Product
  Gain10 : Gain  Gain=-1
  Gain9 : Gain  Gain=-1
  Sum1 : Sum  Inputs=+-
  Sum10 : Sum  Inputs=+-|
  Sum11 : Sum  Inputs=|-+
  Trigonometric Function : Trigonometry  Operator=atan  OutputSignalType=real
  Trigonometric Function1 : Trigonometry  Operator=cos
  Trigonometric Function2 : Trigonometry
  Vx : Outport
  Vy : Outport  Port=2
  wires:
  Kap/1 -> Divide4/2
  VyG/1 -> Sum11/2
  Sum10/1 -> Vx/1  "Vx"
  Sum11/1 -> Vy/1  "Vy"
  VxG/1 -> Sum10/1
  Gain9/1 -> [IFVMoveAngle]
  Sum1/1 -> Divide4/1
  Trigonometric Function2/1 -> Divide11/2
  [IFVMoveAngle] -> Gain10/1
  Divide3/1 -> Sum1/2
  Gain10/1 -> Trigonometric Function2/1, Trigonometric Function1/1
  Divide5/1 -> Sum10/2
  Divide4/1 -> Trigonometric Function/1
  Trigonometric Function1/1 -> Divide5/2
  Constant2/1 -> Sum1/1
  Divide11/1 -> Sum11/1
  Trigonometric Function/1 -> Gain9/1
  Constant4/1 -> Divide3/1
  VxvRef/1 -> Divide3/3, Divide5/1, Divide11/1, Divide3/2

== system Noa_Nofusion/TOS/Subsystem2/ObjMatrixTransit/Subsystem/For Each Subsystem ==
  <EQ4_OBJ_ELEM> : Inport  Partition=on  PartitionDimension=1  PartitionWidth=1  PartitionOffset=0
  Bus Selector : BusSelector  OutputSignals=OBJ_ID,OBJ_Existence_Probability,OBJ_Object_Class,OBJ_Width,OBJ_Long_Distance,OBJ_Lat_Distance,OBJ_Abs_Long_Acc,OBJ_Abs_Long_Velocity,OBJ_Abs_Lat_Velocity,OBJ_Brake_Light,OBJ_Object_Age,OBJ_Motion_Status,OBJ_Motion_Category,OBJ_Motion_Orientation
  For Each : ForEach  DisableCoverage=on
  id : Outport  ConcatenationDimension=1
  confidence : Outport  Port=2  ConcatenationDimension=1
  classification : Outport  Port=3  ConcatenationDimension=1
  width : Outport  Port=4  ConcatenationDimension=1
  LongDis : Outport  Port=5  ConcatenationDimension=1
  LatDis : Outport  Port=6  ConcatenationDimension=1
  AbsLongAcc : Outport  Port=7  ConcatenationDimension=1
  AbsLongVel : Outport  Port=8  ConcatenationDimension=1
  AbsLatVel : Outport  Port=9  ConcatenationDimension=1
  BrakeLight : Outport  Port=10  ConcatenationDimension=1
  Age : Outport  Port=11  ConcatenationDimension=1
  motionSts : Outport  Port=12  ConcatenationDimension=1
  motionCategory : Outport  Port=13  ConcatenationDimension=1
  motionOrientation : Outport  Port=14  ConcatenationDimension=1
  wires:
  <EQ4_OBJ_ELEM>/1 -> Bus Selector/1
  Bus Selector/12 -> motionSts/1  "<OBJ_Motion_Status>"
  Bus Selector/6 -> LatDis/1  "<OBJ_Lat_Distance>"
  Bus Selector/9 -> AbsLatVel/1  "<OBJ_Abs_Lat_Velocity>"
  Bus Selector/7 -> AbsLongAcc/1  "<OBJ_Abs_Long_Acc>"
  Bus Selector/1 -> id/1  "<OBJ_ID>"
  Bus Selector/2 -> confidence/1  "<OBJ_Existence_Probability>"
  Bus Selector/10 -> BrakeLight/1  "<OBJ_Brake_Light>"
  Bus Selector/8 -> AbsLongVel/1  "<OBJ_Abs_Long_Velocity>"
  Bus Selector/5 -> LongDis/1  "<OBJ_Long_Distance>"
  Bus Selector/11 -> Age/1  "<OBJ_Object_Age>"
  Bus Selector/4 -> width/1  "<OBJ_Width>"
  Bus Selector/14 -> motionOrientation/1  "<OBJ_Motion_Orientation>"
  Bus Selector/3 -> classification/1  "<OBJ_Object_Class>"
  Bus Selector/13 -> motionCategory/1  "<OBJ_Motion_Category>"

== system Noa_Nofusion/TOS/Subsystem2/ObjMatrixTransit/Subsystem/For Iterator Subsystem ==
  <EQ4_OBJ_ELEM> : Inport
  Bus Selector : BusSelector  OutputSignals=OBJ_ID,OBJ_Existence_Probability,OBJ_Object_Class,OBJ_Width,OBJ_Long_Distance,OBJ_Lat_Distance,OBJ_Abs_Long_Acc,OBJ_Abs_Long_Velocity,OBJ_Abs_Lat_Velocity,OBJ_Brake_Light,OBJ_Object_Age,OBJ_Motion_Status,OBJ_Motion_Category,OBJ_Motion_Orientation
  For Iterator : ForIterator  IterationLimit=20
  Selector : Selector  InputPortWidth=20  IndexOptions=Index vector (port)  Indices=[1 3]  OutputSizes=1
  id : Outport
  confidence : Outport  Port=2
  classification : Outport  Port=3
  width : Outport  Port=4
  LongDis : Outport  Port=5
  LatDis : Outport  Port=6
  AbsLongAcc : Outport  Port=7
  AbsLongVel : Outport  Port=8
  AbsLatVel : Outport  Port=9
  BrakeLight : Outport  Port=10
  Age : Outport  Port=11
  motionSts : Outport  Port=12
  motionCategory : Outport  Port=13
  motionOrientation : Outport  Port=14
  wires:
  <EQ4_OBJ_ELEM>/1 -> Selector/1
  For Iterator/1 -> Selector/2
  Selector/1 -> Bus Selector/1
  Bus Selector/1 -> id/1  "<OBJ_ID>"
  Bus Selector/2 -> confidence/1  "<OBJ_Existence_Probability>"
  Bus Selector/3 -> classification/1  "<OBJ_Object_Class>"
  Bus Selector/4 -> width/1  "<OBJ_Width>"
  Bus Selector/5 -> LongDis/1  "<OBJ_Long_Distance>"
  Bus Selector/6 -> LatDis/1  "<OBJ_Lat_Distance>"
  Bus Selector/7 -> AbsLongAcc/1  "<OBJ_Abs_Long_Acc>"
  Bus Selector/8 -> AbsLongVel/1  "<OBJ_Abs_Long_Velocity>"
  Bus Selector/9 -> AbsLatVel/1  "<OBJ_Abs_Lat_Velocity>"
  Bus Selector/10 -> BrakeLight/1  "<OBJ_Brake_Light>"
  Bus Selector/11 -> Age/1  "<OBJ_Object_Age>"
  Bus Selector/12 -> motionSts/1  "<OBJ_Motion_Status>"
  Bus Selector/13 -> motionCategory/1  "<OBJ_Motion_Category>"
  Bus Selector/14 -> motionOrientation/1  "<OBJ_Motion_Orientation>"

== system Noa_Nofusion/TOS2/Subsystem1/ACCOSM/HWA_Task100ms1/OTL1 ==
  vRef : Inport
  tCycle : Inport  Port=2
  tSameHandle : Inport  Port=3
  CutIn : Inport  Port=4
  P0Dx : Inport  Port=5
  P0Dy : Inport  Port=6
  EgoDDeltaX : Inport  Port=7
  EgoDDeltaY : Inport  Port=8
  EgoCosOfPsi : Inport  Port=9
  EgoSinOfPsi : Inport  Port=10
  Memory31 : Memory  InitialCondition=zeros(24,1)  InheritSampleTime=on
  Memory32 : Memory  InitialCondition=zeros(24,1)  InheritSampleTime=on
  Memory33 : Memory  InitialCondition=uint8(0)  InheritSampleTime=on
  P0TrajHistCalc01 : MATLAB Function  TreatAsAtomicUnit=on
  P0TrajHistCalc1 : MATLAB Function  TreatAsAtomicUnit=on
  Terminator : Terminator
  Terminator1 : Terminator
  Terminator2 : Terminator
  LineValid : Outport
  a : Outport  Port=2
  b : Outport  Port=3
  c : Outport  Port=4
  d : Outport  Port=5
  dxMin : Outport  Port=6
  dxMax : Outport  Port=7
  wires:
  EgoDDeltaX/1 -> P0TrajHistCalc01/7(EgoDDeltaX)
  P0TrajHistCalc01/3(P0TrajHistDyv) -> P0TrajHistCalc1/3(P0TrajHistDyv1), Memory31/1
  Memory33/1 -> P0TrajHistCalc01/11(P0TrajHistNumK1)
  EgoSinOfPsi/1 -> P0TrajHistCalc01/10(EgoSinOfPsi)
  P0TrajHistCalc01/1(P0TrajHistNum) -> P0TrajHistCalc1/1(P0TrajHistNum1), Memory33/1
  Memory32/1 -> P0TrajHistCalc01/12(P0TrajHistDxvK1)
  P0TrajHistCalc01/2(P0TrajHistDxv) -> P0TrajHistCalc1/2(P0TrajHistDxv1), Memory32/1
  EgoDDeltaY/1 -> P0TrajHistCalc01/8(EgoDDeltaY)
  Memory31/1 -> P0TrajHistCalc01/13(P0TrajHistDyvK1)
  tCycle/1 -> P0TrajHistCalc01/2(tCycle)
  EgoCosOfPsi/1 -> P0TrajHistCalc01/9(EgoCosOfPsi)
  tSameHandle/1 -> P0TrajHistCalc01/3(tSameHandle)
  P0Dx/1 -> P0TrajHistCalc01/5(P0Dx)
  P0Dy/1 -> P0TrajHistCalc01/6(P0Dy)
  P0TrajHistCalc1/1(P0TrajHistNum) -> Terminator/1
  P0TrajHistCalc1/2(P0TrajHistDxv) -> Terminator1/1
  P0TrajHistCalc1/3(P0TrajHistDyv) -> Terminator2/1
  P0TrajHistCalc1/4(LineValid) -> LineValid/1
  P0TrajHistCalc1/5(a) -> a/1
  P0TrajHistCalc1/6(b) -> b/1
  P0TrajHistCalc1/7(c) -> c/1
  P0TrajHistCalc1/9(dxMin) -> dxMin/1
  P0TrajHistCalc1/10(dxMax) -> dxMax/1
  P0TrajHistCalc1/8(d) -> d/1
  CutIn/1 -> P0TrajHistCalc01/4(CutIn)
  vRef/1 -> P0TrajHistCalc01/1(vRef)

== system Noa_Nofusion/TOS2/Subsystem1/ACCOSM/HWA_Task100ms1/Trajectory ==
  Kap : Inport
  VxvRef : Inport  Port=2
  AlpSideSlipAngle : Inport  Port=3
  ObjValid : Inport  Port=4
  ObjDx : Inport  Port=5
  ObjDy : Inport  Port=6
  ObjClass : Inport  Port=7
  ObjCntAlive : Inport  Port=8
  Terminator{1,3..10} (9 alike) : Terminator
  Trajectory : Subsystem  mask{ObjNum=15, TrajNum=10, BufNum=24}
      mask prompts: ObjNum "ObjectNumber"; TrajNum "TrajectoryNumber"; BufNum "BufferNumber"
  Out8 : Outport
  Out9 : Outport  Port=2
  Out10 : Outport  Port=3
  Out11 : Outport  Port=4
  Out12 : Outport  Port=5
  Out13 : Outport  Port=6
  EgoMove : Outport  Port=7
  wires:
  Trajectory/15(TrajHistBufferClass) -> Terminator1/1
  Trajectory/14(TrajHistBufferTTimeStamp) -> Terminator6/1
  Trajectory/9(ObjTrajNumber) -> Out9/1
  Trajectory/3(EgoTrajHistDyv) -> Terminator5/1
  VxvRef/1 -> Trajectory/2(VxvRef)
  Trajectory/4(EgoTrajHistTTimeStamp) -> Terminator7/1
  Trajectory/6(ObjMatrix) -> Terminator10/1
  Trajectory/10(TrajCurrentIndex) -> Out10/1
  Trajectory/7(TrajUsed) -> Terminator9/1
  AlpSideSlipAngle/1 -> Trajectory/3(AlpSideSlipAngle)
  Trajectory/1(EgoTrajHistCurrentIndex) -> Terminator3/1
  Trajectory/5(ObjPrio) -> Terminator8/1
  Trajectory/2(EgoTrajHistDxv) -> Terminator4/1
  Trajectory/8(TrajHistBufferBTrajEnd) -> Out8/1
  Kap/1 -> Trajectory/1(KapTraj)
  ObjCntAlive/1 -> Trajectory/8(ObjectCntAlive)
  ObjClass/1 -> Trajectory/7(ObjectClass)
  ObjDy/1 -> Trajectory/6(ObjectDy)
  ObjDx/1 -> Trajectory/5(ObjectDx)
  ObjValid/1 -> Trajectory/4(ObjValid)
  Trajectory/13(TrajHistBufferDyv) -> Out13/1
  Trajectory/12(TrajHistBufferDxv) -> Out12/1
  Trajectory/11(TrajHistBufferBValid) -> Out11/1
  Trajectory/16(EgoMove) -> EgoMove/1

== system Noa_Nofusion/TOS2/Subsystem1/ACCOSM/HWA_Task100ms1/VxVy ==
  VxvRef : Inport
  Kap : Inport  Port=2
  VxG : Inport  Port=3
  VyG : Inport  Port=4
  Constant2 : Constant  Value=P_Global_EQ2RearAxisX_m  OutDataTypeStr=single
  Constant4 : Constant  Value=SideSlipAnglefactor  OutDataTypeStr=single
  Divide11 : Product
  Divide3 : Product  Inputs=3
  Divide4 : Product
  Divide5 : Product
  Gain10 : Gain  Gain=-1
  Gain9 : Gain  Gain=-1
  Sum1 : Sum  Inputs=+-
  Sum10 : Sum  Inputs=+-|
  Sum11 : Sum  Inputs=|-+
  Trigonometric Function : Trigonometry  Operator=atan  OutputSignalType=real
  Trigonometric Function1 : Trigonometry  Operator=cos
  Trigonometric Function2 : Trigonometry
  Vx : Outport
  Vy : Outport  Port=2
  wires:
  Kap/1 -> Divide4/2
  VyG/1 -> Sum11/2
  Sum10/1 -> Vx/1  "Vx"
  Sum11/1 -> Vy/1  "Vy"
  VxG/1 -> Sum10/1
  Gain9/1 -> [IFVMoveAngle]
  Sum1/1 -> Divide4/1
  Trigonometric Function2/1 -> Divide11/2
  [IFVMoveAngle] -> Gain10/1
  Divide3/1 -> Sum1/2
  Gain10/1 -> Trigonometric Function2/1, Trigonometric Function1/1
  Divide5/1 -> Sum10/2
  Divide4/1 -> Trigonometric Function/1
  Trigonometric Function1/1 -> Divide5/2
  Constant2/1 -> Sum1/1
  Divide11/1 -> Sum11/1
  Trigonometric Function/1 -> Gain9/1
  Constant4/1 -> Divide3/1
  VxvRef/1 -> Divide3/3, Divide5/1, Divide11/1, Divide3/2

== system Noa_Nofusion/TOS2/Subsystem1/ACCOSM/ObjMatrixTransit/Subsystem ==
  Count : Inport
  <EQ4_OBJ_ELEM> : Inport  Port=2
  Bus Creator : BusCreator  Inputs=12
  Bus Selector : BusSelector  OutputSignals=id,BrakeLight,classification,LatDis,AbsLatVel,AbsLongAcc,LongDis,AbsLongVel,width,Age,motionSts
  For Each Subsystem : Subsystem  TreatAsAtomicUnit=on
  For Iterator Subsystem : Subsystem  Commented=on  TreatAsAtomicUnit=on
  MATLAB Function1 : MATLAB Function  TreatAsAtomicUnit=on
  Obj : Stateflow chart  Commented=on  TreatAsAtomicUnit=on
  Terminator : Terminator
  Terminator1 : Terminator
  Unit Delay1 : UnitDelay  SampleTime=-1  HasFrameUpgradeWarning=on
  ObjID : Outport
  ObjValid : Outport  Port=2
  ObjBrakeLightIndic : Outport  Port=3
  ObjClassification : Outport  Port=4
  ObjLatPos : Outport  Port=5
  ObjLatVel : Outport  Port=6
  ObjLongAccel : Outport  Port=7
  ObjLongVel : Outport  Port=8
  ObjWidth : Outport  Port=9
  ObjCnt : Outport  Port=10
  ObjMoveSts : Outport  Port=11
  ObjLongPos : Outport  Port=12
  P : Outport  Port=13
  wires:
  For Each Subsystem/6(LatDis) -> Bus Creator/6  "LatDis"
  Bus Creator/1 -> Bus Selector/1
  MATLAB Function1/13(ObjID) -> ObjID/1, Unit Delay1/1  "ObjBrakeLightIndic"
  For Each Subsystem/10(BrakeLight) -> Bus Creator/10  "BrakeLight"
  MATLAB Function1/5(ObjLatPos) -> ObjLatPos/1
  For Each Subsystem/7(AbsLongAcc) -> Bus Creator/7  "AbsLongAcc"
  For Each Subsystem/12(motionSts) -> Bus Creator/12  "motionSts"
  MATLAB Function1/4(ObjClassification) -> ObjClassification/1
  MATLAB Function1/7(ObjLongAccel) -> ObjLongAccel/1
  For Each Subsystem/14(motionOrientation) -> Terminator1/1
  Count/1 -> MATLAB Function1/1(Count)
  For Each Subsystem/8(AbsLongVel) -> Bus Creator/8  "AbsLongVel"
  For Each Subsystem/4(width) -> Bus Creator/4  "width"
  For Each Subsystem/13(motionCategory) -> Terminator/1
  For Each Subsystem/9(AbsLatVel) -> Bus Creator/9  "AbsLatVel"
  For Each Subsystem/5(LongDis) -> Bus Creator/5  "LongDis"
  Bus Selector/10 -> MATLAB Function1/11(Age)  "<Age>"
  For Each Subsystem/3(classification) -> Bus Creator/3  "classification"
  Bus Selector/8 -> MATLAB Function1/9(LongVel)  "<AbsLongVel>"
  Bus Selector/3 -> MATLAB Function1/4(Class)  "<classification>"
  For Each Subsystem/1(id) -> Bus Creator/1  "id"
  For Each Subsystem/11(Age) -> Bus Creator/11  "Age"
  For Each Subsystem/2(confidence) -> Bus Creator/2  "confidence"
  Bus Selector/7 -> MATLAB Function1/8(LongDis)  "<LongDis>"
  Bus Selector/9 -> MATLAB Function1/10(Width)  "<width>"
  Bus Selector/5 -> MATLAB Function1/6(LatVel)  "<AbsLatVel>"
  Bus Selector/6 -> MATLAB Function1/7(LongAccel)  "<AbsLongAcc>"
  Bus Selector/4 -> MATLAB Function1/5(LatDis)  "<LatDis>"
  MATLAB Function1/11(ObjMoveSts) -> ObjMoveSts/1
  Bus Selector/11 -> MATLAB Function1/12(MotionSts)  "<motionSts>"
  MATLAB Function1/12(ObjLongPos) -> ObjLongPos/1
  MATLAB Function1/1(P) -> P/1
  Bus Selector/2 -> MATLAB Function1/3(BrakeLight_b)  "<BrakeLight>"
  Bus Selector/1 -> MATLAB Function1/2(ID)  "<id>"
  Unit Delay1/1 -> MATLAB Function1/13(ObjIDK1)
  <EQ4_OBJ_ELEM>/1 -> For Each Subsystem/1(<EQ4_OBJ_ELEM>)
  MATLAB Function1/2(ObjValid) -> ObjValid/1
  MATLAB Function1/6(ObjLatVel) -> ObjLatVel/1
  MATLAB Function1/3(ObjBrakeLightIndic) -> ObjBrakeLightIndic/1
  MATLAB Function1/8(ObjLongVel) -> ObjLongVel/1
  MATLAB Function1/9(ObjWidth) -> ObjWidth/1
  MATLAB Function1/10(ObjCnt) -> ObjCnt/1
